simulink model "encode2"  (R2024b)
settings: Solver=FixedStepAuto  StartTime=0.0  StopTime=inf  FixedStep=0.01  RelTol=1e-3  EnableMultiTasking=on
libraries: simulink x6, stm32f4xxblockslib x5, stm32g4xxblockslib x3
settings Model: STM32="{\"EncoderBlockForG4\":[{\"ID\":\"encode:1\"},{\"ID\":\"encode:52\"},{\"ID\":\"encode:72\"}],\"DigitalPortRead\":[{\"ID\":\"encode:8\"},{\"ID\":\"encode:7\"},{\"ID\":\"encode:25\"},{\"ID\":\"encode:165\"},{\"ID\":\"encode:176\"}]}"  Creator=A1nz_01  LastModifiedBy=A1nz_01
settings OptimizationCC: DefaultParameterBehavior=Inlined  EnhancedBackFolding=on  PassReuseOutputArgsAs=Individual arguments  ZeroExternalMemoryAtStartup=off  ZeroInternalMemoryAtStartup=off  MaxStackSize=512  OptimizeBlockOrder=speed  DifferentSizesBufferReuse=on  OptimizationCustomize=off  EfficientTunableParamExpr=on
settings DebuggingCC: ParameterTunabilityLossMsg=error
settings HardwareCC: ProdBitPerPointer=32  ProdBitPerSizeT=32  ProdBitPerPtrDiffT=32  ProdLargestAtomicInteger=Long  ProdLargestAtomicFloat=Double  ProdWordSize=32  ProdLongLongMode=on  ProdHWDeviceType=ARM Compatible->ARM Cortex-M
settings SFSimCC: MATLABDynamicMemAlloc=off
settings RTWCC: Description=Embedded Coder  SystemTargetFile=ert.tlc  HardwareBoard=STM32G4xx Based  TemplateMakefile=ert_default_tmf  Toolchain=GNU Tools for ARM Embedded Processors
settings CodeAppCC: ForceParamTrailComments=on  IgnoreCustomStorageClasses=off  OperatorAnnotations=on  SimulinkDataObjDesc=on  SFDataObjDesc=on  InsertBlockDesc=on
settings ERTTargetCC: TargetLangStandard=C99 (ISO)  CodeReplacementLibrary=ARM Cortex-M  ExtModeTransport=3  ExtModeStaticAlloc=on  ExtModeStaticAllocSize=2048  ExtModeMexFile=ext_xcp  ExtModeIntrfLevel=Level2 - Open

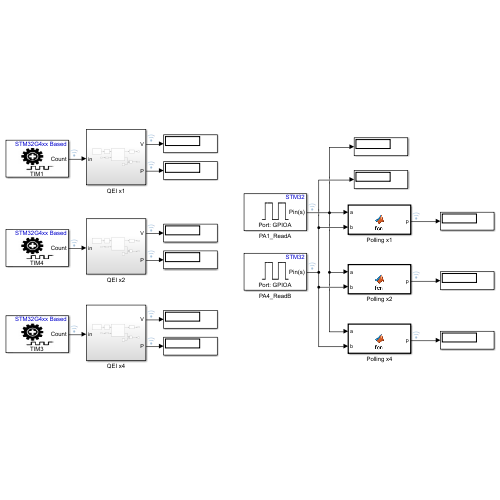
[thumbnail: Simulink's stored preview of the top-level diagram]
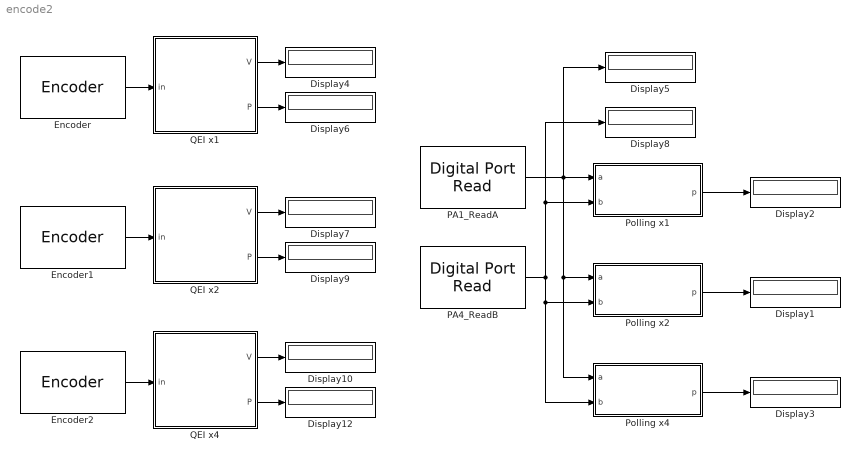
== system encode2 ==
  Display{1..10,12} (11 alike) : Display
  Encoder : stm32g4xxblockslib/Encoder  TimerModule=TIM1  EnableResetInput=off  OutputCountAfterFirstIndex=off  OutputValidIndex=off  OutputDirection=off  OutputStatus=off  SampleTime=-1
  Encoder1 : stm32g4xxblockslib/Encoder  TimerModule=TIM4  EnableResetInput=off  OutputCountAfterFirstIndex=off  OutputValidIndex=off  OutputDirection=off  OutputStatus=off  SampleTime=-1
  Encoder2 : stm32g4xxblockslib/Encoder  TimerModule=TIM3  EnableResetInput=off  OutputCountAfterFirstIndex=off  OutputValidIndex=off  OutputDirection=off  OutputStatus=off  SampleTime=-1
  PA1_ReadA : stm32f4xxblockslib/Digital Port Read  PortName=GPIOA  PinNumber=[1]  ReadOperation=on  IOAsArray=on  SampleTime=-1  EnableSimPort=off  hoistedMaskSrc=ECSoC/ECSimCodegen/Digital Port Read
      settings: LibrarySourceBlock=stm32g4xxblockslib/Digital Port Read
  PA4_ReadB : stm32f4xxblockslib/Digital Port Read  PortName=GPIOA  PinNumber=[4]  ReadOperation=on  IOAsArray=on  SampleTime=-1  EnableSimPort=off  hoistedMaskSrc=ECSoC/ECSimCodegen/Digital Port Read
      settings: LibrarySourceBlock=stm32g4xxblockslib/Digital Port Read
  Polling x1 : MATLAB Function  TreatAsAtomicUnit=on
  Polling x2 : MATLAB Function  TreatAsAtomicUnit=on
  Polling x4 : MATLAB Function  TreatAsAtomicUnit=on
  QEI x1 : Subsystem
  QEI x2 : Subsystem
  QEI x4 : Subsystem
  wires:
  PA4_ReadB/1 -> Polling x2/2(b), Polling x4/2(b), Display8/1, Polling x1/2(b)
  PA1_ReadA/1 -> Display5/1, Polling x4/1(a), Polling x2/1(a), Polling x1/1(a)
  Encoder/1 -> QEI x1/1(in)
  QEI x1/1(V) -> Display4/1
  QEI x1/2(P) -> Display6/1
  QEI x2/2(P) -> Display9/1
  QEI x2/1(V) -> Display7/1
  Encoder1/1 -> QEI x2/1(in)
  QEI x4/2(P) -> Display12/1
  QEI x4/1(V) -> Display10/1
  Encoder2/1 -> QEI x4/1(in)
  Polling x1/1(p) -> Display2/1
  Polling x2/1(p) -> Display1/1
  Polling x4/1(p) -> Display3/1

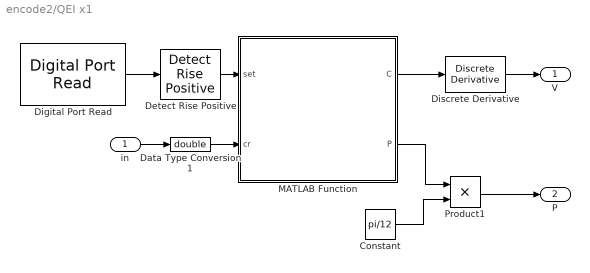
== system encode2/QEI x1 ==
  in : Inport
  Constant : Constant  Value=pi/12
  Data Type Conversion1 : DataTypeConversion  OutDataTypeStr=double  SaturateOnIntegerOverflow=off  RndMeth=Floor
  Detect Rise Positive : simulink/Logic and Bit Operations/Detect Rise Positive  vinit=0  OutDataTypeStr=boolean
  Digital Port Read : stm32f4xxblockslib/Digital Port Read  PortName=GPIOC  PinNumber=[13]  ReadOperation=on  IOAsArray=on  SampleTime=-1  EnableSimPort=off  hoistedMaskSrc=ECSoC/ECSimCodegen/Digital Port Read
      settings: LibrarySourceBlock=stm32g4xxblockslib/Digital Port Read
  Discrete Derivative : simulink/Discrete/Discrete Derivative  gainval=1.0  ICPrevScaledInput=0.0  OutMin=[]  OutMax=[]  OutDataType=fixdt(1, 16)  OutScaling=2^-10  DoSatur=off
  MATLAB Function : MATLAB Function  TreatAsAtomicUnit=on
  Product1 : Product
  V : Outport
  P : Outport  Port=2
  wires:
  Digital Port Read/1 -> Detect Rise Positive/1
  Detect Rise Positive/1 -> MATLAB Function/1(set)
  Data Type Conversion1/1 -> MATLAB Function/2(cr)
  in/1 -> Data Type Conversion1/1
  MATLAB Function/1(C) -> Discrete Derivative/1
  Discrete Derivative/1 -> V/1
  MATLAB Function/2(P) -> Product1/1
  Constant/1 -> Product1/2
  Product1/1 -> P/1

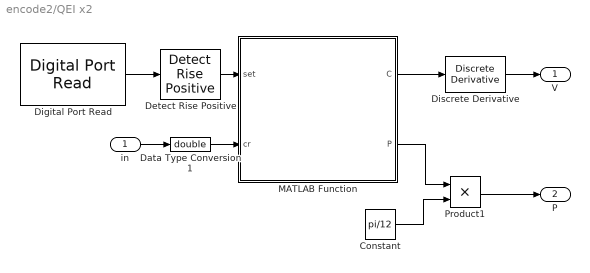
== system encode2/QEI x2 ==
  in : Inport
  Constant : Constant  Value=pi/12
  Data Type Conversion1 : DataTypeConversion  OutDataTypeStr=double  SaturateOnIntegerOverflow=off  RndMeth=Floor
  Detect Rise Positive : simulink/Logic and Bit Operations/Detect Rise Positive  vinit=0  OutDataTypeStr=boolean
  Digital Port Read : stm32f4xxblockslib/Digital Port Read  PortName=GPIOC  PinNumber=[13]  ReadOperation=on  IOAsArray=on  SampleTime=-1  EnableSimPort=off  hoistedMaskSrc=ECSoC/ECSimCodegen/Digital Port Read
  Discrete Derivative : simulink/Discrete/Discrete Derivative  gainval=1.0  ICPrevScaledInput=0.0  OutMin=[]  OutMax=[]  OutDataType=fixdt(1, 16)  OutScaling=2^-10  DoSatur=off
  MATLAB Function : MATLAB Function  TreatAsAtomicUnit=on
  Product1 : Product
  V : Outport
  P : Outport  Port=2
  wires:
  Digital Port Read/1 -> Detect Rise Positive/1
  Detect Rise Positive/1 -> MATLAB Function/1(set)
  Data Type Conversion1/1 -> MATLAB Function/2(cr)
  in/1 -> Data Type Conversion1/1
  MATLAB Function/1(C) -> Discrete Derivative/1
  Discrete Derivative/1 -> V/1
  MATLAB Function/2(P) -> Product1/1
  Constant/1 -> Product1/2
  Product1/1 -> P/1

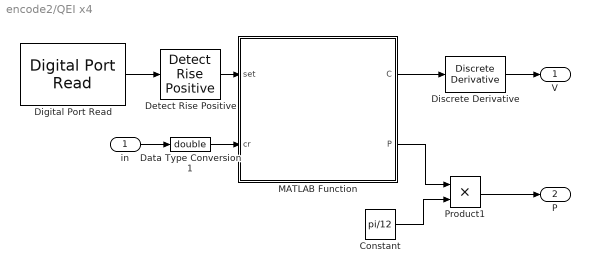
== system encode2/QEI x4 ==
  in : Inport
  Constant : Constant  Value=pi/12
  Data Type Conversion1 : DataTypeConversion  OutDataTypeStr=double  SaturateOnIntegerOverflow=off  RndMeth=Floor
  Detect Rise Positive : simulink/Logic and Bit Operations/Detect Rise Positive  vinit=0  OutDataTypeStr=boolean
  Digital Port Read : stm32f4xxblockslib/Digital Port Read  PortName=GPIOC  PinNumber=[13]  ReadOperation=on  IOAsArray=on  SampleTime=-1  EnableSimPort=off  hoistedMaskSrc=ECSoC/ECSimCodegen/Digital Port Read
  Discrete Derivative : simulink/Discrete/Discrete Derivative  gainval=1.0  ICPrevScaledInput=0.0  OutMin=[]  OutMax=[]  OutDataType=fixdt(1, 16)  OutScaling=2^-10  DoSatur=off
  MATLAB Function : MATLAB Function  TreatAsAtomicUnit=on
  Product1 : Product
  V : Outport
  P : Outport  Port=2
  wires:
  Digital Port Read/1 -> Detect Rise Positive/1
  Detect Rise Positive/1 -> MATLAB Function/1(set)
  Data Type Conversion1/1 -> MATLAB Function/2(cr)
  in/1 -> Data Type Conversion1/1
  MATLAB Function/1(C) -> Discrete Derivative/1
  Discrete Derivative/1 -> V/1
  MATLAB Function/2(P) -> Product1/1
  Constant/1 -> Product1/2
  Product1/1 -> P/1

== matlab function encode2/Polling x2 ==
  data: a input; p output; b input
function p = fcn(a,b)
    persistent pos;
    persistent trig;
    if isempty(trig)
        trig = 1;
        pos = 0;
    end
    if a-b == -1 && trig
        pos = pos + 1;
        trig = 2;
    elseif a-b == 1 && trig
        pos = pos -1;
        trig = 2;
    end

    if a == 0 && b == 0 
        trig = 0;
    end

    if a-b == 1 && trig == 0
        pos = pos + 1;
        trig = -1;
    elseif a-b == -1 && trig == 0
        pos = pos -1;
        trig = 1;
    end

    if a == 1 && b == 1
        trig = 1;
    end
    p = pos;
end

== matlab function encode2/Polling x1 ==
  data: a input; p output; b input
function p = fcn(a,b)
    persistent pos;
    persistent trig;
    if isempty(trig)
        trig = 1;
        pos = 0;
    end
    if a-b == -1 && trig
        pos = pos + 1;
        trig = 0;
    elseif a-b == 1 && trig
        pos = pos -1;
        trig = 0;
    end

    if a == 1 && b == 1
        trig = 1;
    end
    p = pos;
end

== matlab function encode2/Polling x4 ==
  data: a input; p output; b input
function p = fcn(a,b)
    persistent pos;
    persistent trigA;
    persistent trigB;
    if isempty(trigA)
        trigA = 1;
        trigB = 1;
        pos = 0;
    end
    if a-b == -1 && trigA
        pos = pos + 1;
        trigA = 2;
    elseif a-b == 1 && trigA
        pos = pos -1;
        trigA = 2;
    end


    if a-b == -1 && trigA == 0
        pos = pos + 1;
        trigA = -1;
    elseif a-b == 1 && trigA == 0
        pos = pos -1;
        trigA = -1;
    end


    if b-a == 1 && trigB
        pos = pos + 1;
        trigB = 2;
    elseif b-a == -1 && trigB
        pos = pos - 1;
        trigB = 2;
    end

    if b-a == 1 && trigB == 0
        pos = pos + 1;
        trigB = -1;
    elseif b-a == -1 && trigB == 0
        pos = pos - 1;
        trigB = -1;
    end

    if a == 0 && b == 0
        trigA = 0;
        trigB = 0;
    end

    if a == 1 && b == 1
        trigA = 1;
        trigB = 1;
    end
    p = pos;
end

== matlab function encode2/QEI x1/MATLAB Function ==
  data: C output; P output; set input; cr input
function [C,P] = fcn(set,cr)
    persistent pr;
    persistent hom;
    persistent ps;
    max = 2048;

    if isempty(pr)
        pr = cr;
        hom = 0;
        ps = 0;
    end

    delta = cr - pr;

    if delta <= -1*(max/2)
        delta = delta + max + 1;
    elseif delta >= max/2
        delta = delta -max - 1;
    end

    if set
        hom = ps;
    end
    ps = ps + delta;
    C = ps - hom;
    pr = cr;
    P = C;
end

== matlab function encode2/QEI x2/MATLAB Function ==
  data: C output; P output; set input; cr input
function [C,P] = fcn(set,cr)
    persistent pr;
    persistent hom;
    persistent ps;
    max = 2048;

    if isempty(pr)
        pr = cr;
        hom = 0;
        ps = 0;
    end

    delta = cr - pr;

    if delta <= -1*(max/2)
        delta = delta + max + 1;
    elseif delta >= max/2
        delta = delta -max - 1;
    end

    if set
        hom = ps;
    end
    ps = ps + delta;
    C = ps - hom;
    pr = cr;
    P = C;
end

== matlab function encode2/QEI x4/MATLAB Function ==
  data: C output; P output; set input; cr input
function [C,P] = fcn(set,cr)
    persistent pr;
    persistent hom;
    persistent ps;
    max = 2048;

    if isempty(pr)
        pr = cr;
        hom = 0;
        ps = 0;
    end

    delta = cr - pr;

    if delta <= -1*(max/2)
        delta = delta + max + 1;
    elseif delta >= max/2
        delta = delta -max - 1;
    end

    if set
        hom = ps;
    end
    ps = ps + delta;
    C = ps - hom;
    pr = cr;
    P = C;
end
